simulink model "main"  (R2018a)
settings: Solver=VariableStepAuto  StartTime=0.0  StopTime=25  RelTol=1e-3
values from neighbouring files (symbols this model uses):
  g = 9.8    [value.m]
settings Model: Creator=admin  LastModifiedBy=admin

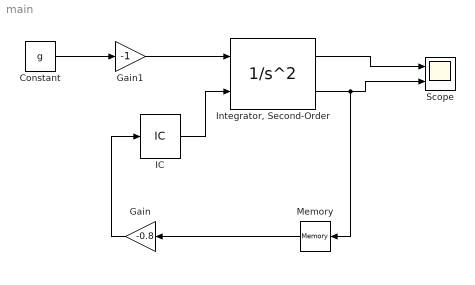
== system main ==
  Constant : Constant  Value=g
  Gain : Gain  Gain=-0.8
  Gain1 : Gain  Gain=-1
  IC : InitialCondition  Value=15
  "Integrator, Second-Order" : SecondOrderIntegrator  ICX=10  LimitX=on  LowerLimitX=0  ICSourceDXDT=external  ReinitDXDTwhenXreachesSaturation=on
  Memory : Memory
  Scope : Scope  NumInputPorts=2
  wires:
  Constant/1 -> Gain1/1
  "Integrator, Second-Order"/1 -> Scope/1
  "Integrator, Second-Order"/2 -> Memory/1, Scope/2
  Memory/1 -> Gain/1
  Gain/1 -> IC/1
  IC/1 -> "Integrator, Second-Order"/2
  Gain1/1 -> "Integrator, Second-Order"/1
